simulink model "control"  (R2014b)
settings: Solver=ode45  StartTime=0.0  StopTime=10  RelTol=1e-5  AbsTol=1e-5
values from neighbouring files (symbols this model uses):
  B_eq = 0    [data.m]
  F1 = lqr(A1,B1,Q,R,N)    [data.m]
  F2 = lqr(A2,B2,Q,R,N)    [data.m]
  F3 = lqr(A3,B3,Q,R,N)    [data.m]
  F4 = lqr(A4,B4,Q,R,N)    [data.m]
  F5 = lqr(A5,B5,Q,R,N)    [data.m]
  F6 = lqr(A6,B6,Q,R,N)    [data.m]
  F7 = lqr(A7,B7,Q,R,N)    [data.m]
  F8 = lqr(A8,B8,Q,R,N)    [data.m]
  F9 = lqr(A9,B9,Q,R,N)    [data.m]
  g = 9.81    [data.m]
  initial = pi/2    (= 1.57079632679)    [data.m]
  J_eq = 1.23e-4    (= 0.000123)    [data.m]
  J_p = 1.20e-4    (= 0.00012)    [data.m]
  K_m = K_t    (= 0.028)    [data.m]
  K_t = 0.028    [data.m]
  K_w = 2.3    [data.m]
  l_p = 0.191    [data.m]
  m = 0.027    [data.m]
  r = 0.0826    [data.m]
  R_m = 3.3    [data.m]
libraries: fuzblock x16
settings Model: Creator=Karol  LastModifiedBy=Aramil_2
settings DataIOCC: SignalLoggingSaveFormat=ModelDataLogs
settings OptimizationCC: ExpressionDepthLimit=2147483647
settings DebuggingCC: UnderspecifiedInitializationDetection=Classic  MergeDetectMultiDrivingBlocksExec=none  FcnCallInpInsideContextMsg=UseLocalSettings  StateNameClashWarn=warning
settings GRTTargetCC: CombineOutputUpdateFcns=off  GRTInterface=on

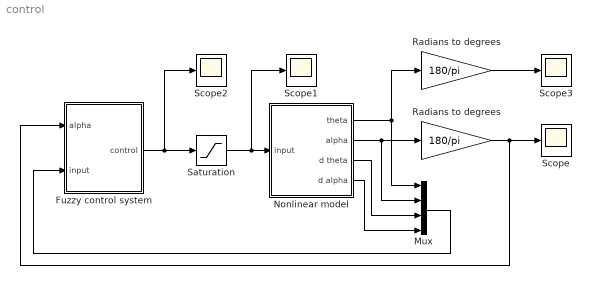
== system control ==
  Fuzzy control system : Subsystem
  Mux : Mux
  "Nonlinear model " : Subsystem
  Radians to degrees : Gain  Gain=180/pi
  "Radians to degrees " : Gain  Gain=180/pi
  Saturation : Saturate  UpperLimit=10  LowerLimit=-10
  Scope{,1..3} (4 alike) : Scope
      Scope settings: YMin=220  YMax=360
      Scope1 settings: TimeRange=20  YMin=0.5375  YMax=0.585
      Scope2 settings: YMin=0.5375  YMax=0.585  SaveName=ScopeData2
      Scope3 settings: TimeRange=5  SaveName=ScopeData3
  wires:
  "Nonlinear model "/2(alpha) -> "Radians to degrees "/1, Mux/2
  "Radians to degrees "/1 -> Scope/1, Fuzzy control system/1(alpha)
  "Nonlinear model "/1(theta) -> Radians to degrees/1, Mux/1
  Mux/1 -> Fuzzy control system/2(input)
  Fuzzy control system/1(control) -> Scope2/1, Saturation/1
  Saturation/1 -> "Nonlinear model "/1(input), Scope1/1
  Radians to degrees/1 -> Scope3/1
  "Nonlinear model "/3(d theta) -> Mux/3
  "Nonlinear model "/4(d alpha) -> Mux/4

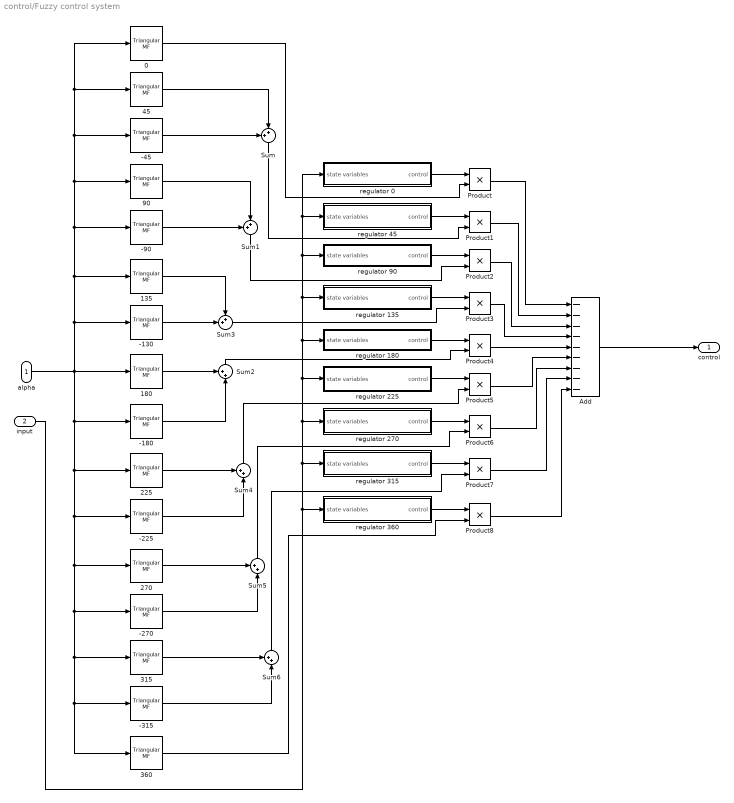
== system control/Fuzzy control system ==
  alpha : Inport
  input : Inport  Port=2
  -130 : fuzblock/Membership  Functions/Triangular MF  a=-180  b=-125  c=-90
  -180 : fuzblock/Membership  Functions/Triangular MF  a=-225  b=-180  c=-130
  -225 : fuzblock/Membership  Functions/Triangular MF  a=-270  b=-225  c=-180
  -270 : fuzblock/Membership  Functions/Triangular MF  a=-315  b=-270  c=-225
  -315 : fuzblock/Membership  Functions/Triangular MF  a=0  b=-315  c=-280
  -45 : fuzblock/Membership  Functions/Triangular MF  a=-90  b=-45  c=0
  -90 : fuzblock/Membership  Functions/Triangular MF  a=-130  b=-90  c=-45
  0 : fuzblock/Membership  Functions/Triangular MF  a=-90  b=0  c=90
  135 : fuzblock/Membership  Functions/Triangular MF  a=90  b=135  c=180
  180 : fuzblock/Membership  Functions/Triangular MF  a=130  b=180  c=225
  225 : fuzblock/Membership  Functions/Triangular MF  a=180  b=225  c=270
  270 : fuzblock/Membership  Functions/Triangular MF  a=225  b=270  c=315
  315 : fuzblock/Membership  Functions/Triangular MF  a=270  b=315  c=360
  360 : fuzblock/Membership  Functions/Triangular MF  a=270  b=360  c=450
  45 : fuzblock/Membership  Functions/Triangular MF  a=0  b=45  c=90
  90 : fuzblock/Membership  Functions/Triangular MF  a=45  b=90  c=130
  Add : Sum  Inputs=---------
  Product{,1..8} (9 alike) : Product  RndMeth=Zero
  Sum{,1..6} (7 alike) : Sum  Inputs=++|
  regulator 0 : Subsystem
  regulator 135 : Subsystem
  regulator 180 : Subsystem
  regulator 225 : Subsystem
  regulator 270 : Subsystem
  regulator 315 : Subsystem
  regulator 360 : Subsystem
  regulator 45 : Subsystem
  regulator 90 : Subsystem
  control : Outport
  wires:
  regulator 0/1(control) -> Product/1
  regulator 45/1(control) -> Product1/1
  regulator 90/1(control) -> Product2/1
  regulator 135/1(control) -> Product3/1
  regulator 180/1(control) -> Product4/1
  regulator 225/1(control) -> Product5/1
  regulator 270/1(control) -> Product6/1
  regulator 315/1(control) -> Product7/1
  regulator 360/1(control) -> Product8/1
  Add/1 -> control/1
  Product/1 -> Add/1
  Product1/1 -> Add/2
  Product2/1 -> Add/3
  Product3/1 -> Add/4
  Product4/1 -> Add/5
  Product5/1 -> Add/6
  Product6/1 -> Add/7
  Product7/1 -> Add/8
  Product8/1 -> Add/9
  0/1 -> Product/2
  Sum/1 -> Product1/2
  Sum1/1 -> Product2/2
  input/1 -> regulator 180/1(state variables), regulator 135/1(state variables), regulator 0/1(state variables), regulator 45/1(state variables), regulator 90/1(state variables), regulator 225/1(state variables), regulator 270/1(state variables), regulator 315/1(state variables), regulator 360/1(state variables)
  45/1 -> Sum/2
  -45/1 -> Sum/1
  90/1 -> Sum1/2
  -90/1 -> Sum1/1
  Sum2/1 -> Product4/2
  Sum3/1 -> Product3/2
  225/1 -> Sum4/1
  -225/1 -> Sum4/2
  315/1 -> Sum6/1
  -315/1 -> Sum6/2
  alpha/1 -> 360/1, -315/1, 315/1, -270/1, 270/1, -225/1, 225/1, -180/1, -90/1, 90/1, 0/1, 45/1, -45/1, 135/1, -130/1, 180/1
  360/1 -> Product8/2
  Sum4/1 -> Product5/2
  Sum5/1 -> Product6/2
  Sum6/1 -> Product7/2
  135/1 -> Sum3/1
  -130/1 -> Sum3/2
  180/1 -> Sum2/1
  -180/1 -> Sum2/2
  270/1 -> Sum5/1
  -270/1 -> Sum5/2

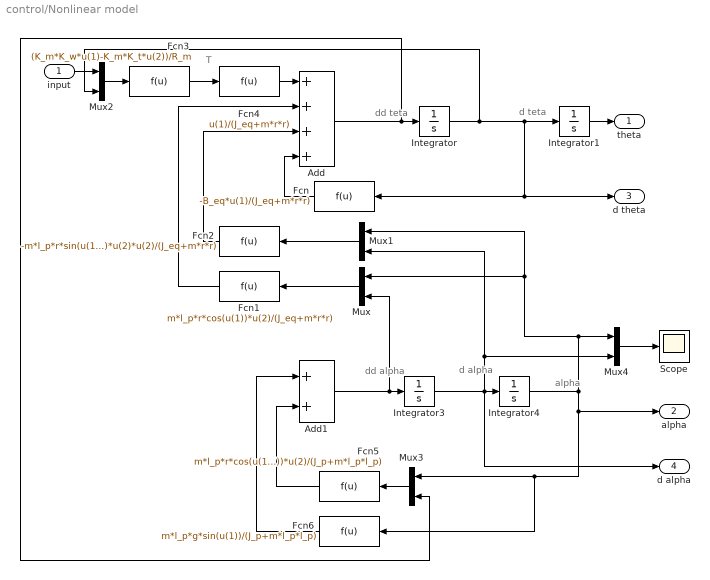
== system control/Nonlinear model  ==
  note: dd teta
  note: d teta
  note: dd alpha
  note: d alpha
  note: alpha
  note: T
  input : Inport
  Add : Sum  Inputs=++++
  Add1 : Sum
  Fcn : Fcn  Expr=-B_eq*u(1)/(J_eq+m*r*r)
  Fcn1 : Fcn  Expr=m*l_p*r*cos(u(1))*u(2)/(J_eq+m*r*r)
  Fcn2 : Fcn  Expr=-m*l_p*r*sin(u(1))*u(2)*u(2)/(J_eq+m*r*r)
  Fcn3 : Fcn  Expr=(K_m*K_w*u(1)-K_m*K_t*u(2))/R_m
  Fcn4 : Fcn  Expr=u(1)/(J_eq+m*r*r)
  Fcn5 : Fcn  Expr=m*l_p*r*cos(u(1))*u(2)/(J_p+m*l_p*l_p)
  Fcn6 : Fcn  Expr=m*l_p*g*sin(u(1))/(J_p+m*l_p*l_p)
  Integrator : Integrator
  Integrator1 : Integrator
  Integrator3 : Integrator
  Integrator4 : Integrator  InitialCondition=initial
  Mux{,1..4} (5 alike) : Mux  Inputs=2
  Scope : Scope
      settings: SaveName=ScopeData7
  theta : Outport
  alpha : Outport  Port=2
  d theta : Outport  Port=3
  d alpha : Outport  Port=4
  wires:
  Add/1 -> Integrator/1, Mux3/2
  Integrator/1 -> Mux2/2, d theta/1, Fcn/1, Integrator1/1
  Add1/1 -> Integrator3/1, Mux/2
  Integrator3/1 -> d alpha/1, Integrator4/1, Mux4/2, Mux1/2
  Integrator4/1 -> Fcn6/1, Mux3/1, alpha/1, Mux/1, Mux1/1, Mux4/1
  Mux/1 -> Fcn1/1
  Mux1/1 -> Fcn2/1
  Mux2/1 -> Fcn3/1
  Fcn3/1 -> Fcn4/1
  Fcn4/1 -> Add/1
  Fcn/1 -> Add/4
  Fcn2/1 -> Add/3
  Fcn1/1 -> Add/2
  Mux3/1 -> Fcn5/1
  Fcn5/1 -> Add1/2
  Fcn6/1 -> Add1/1
  Integrator1/1 -> theta/1
  Mux4/1 -> Scope/1
  input/1 -> Mux2/1

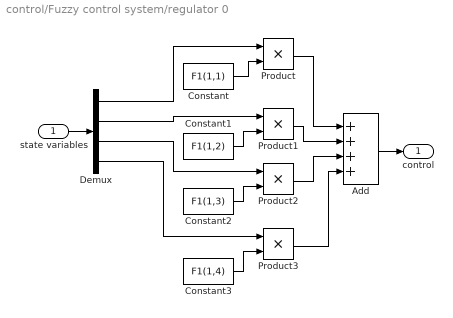
== system control/Fuzzy control system/regulator 0 ==
  state variables : Inport
  Add : Sum  Inputs=++++
  Constant : Constant  Value=F1(1,1)
  Constant1 : Constant  Value=F1(1,2)
  Constant2 : Constant  Value=F1(1,3)
  Constant3 : Constant  Value=F1(1,4)
  Demux : Demux
  Product{,1..3} (4 alike) : Product  RndMeth=Zero
  control : Outport
  wires:
  Demux/1 -> Product/1
  Constant/1 -> Product/2
  Constant1/1 -> Product1/2
  Demux/2 -> Product1/1
  Constant2/1 -> Product2/2
  Demux/3 -> Product2/1
  Constant3/1 -> Product3/2
  Demux/4 -> Product3/1
  Product/1 -> Add/1
  Product1/1 -> Add/2
  Product2/1 -> Add/3
  Product3/1 -> Add/4
  state variables/1 -> Demux/1
  Add/1 -> control/1

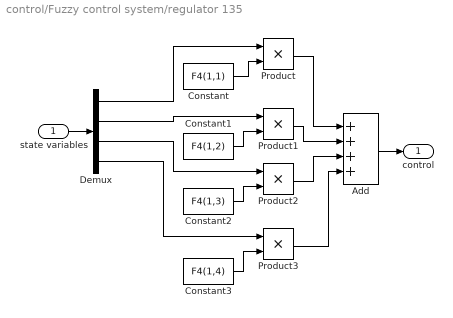
== system control/Fuzzy control system/regulator 135 ==
  state variables : Inport
  Add : Sum  Inputs=++++
  Constant : Constant  Value=F4(1,1)
  Constant1 : Constant  Value=F4(1,2)
  Constant2 : Constant  Value=F4(1,3)
  Constant3 : Constant  Value=F4(1,4)
  Demux : Demux
  Product{,1..3} (4 alike) : Product  RndMeth=Zero
  control : Outport
  wires:
  Add/1 -> control/1
  state variables/1 -> Demux/1
  Product3/1 -> Add/4
  Product2/1 -> Add/3
  Product1/1 -> Add/2
  Product/1 -> Add/1
  Demux/4 -> Product3/1
  Constant3/1 -> Product3/2
  Demux/3 -> Product2/1
  Constant2/1 -> Product2/2
  Demux/2 -> Product1/1
  Constant1/1 -> Product1/2
  Constant/1 -> Product/2
  Demux/1 -> Product/1

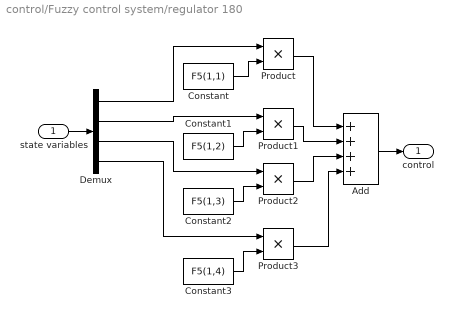
== system control/Fuzzy control system/regulator 180 ==
  state variables : Inport
  Add : Sum  Inputs=++++
  Constant : Constant  Value=F5(1,1)
  Constant1 : Constant  Value=F5(1,2)
  Constant2 : Constant  Value=F5(1,3)
  Constant3 : Constant  Value=F5(1,4)
  Demux : Demux
  Product{,1..3} (4 alike) : Product  RndMeth=Zero
  control : Outport
  wires:
  Demux/1 -> Product/1
  Constant/1 -> Product/2
  Constant1/1 -> Product1/2
  Demux/2 -> Product1/1
  Constant2/1 -> Product2/2
  Demux/3 -> Product2/1
  Constant3/1 -> Product3/2
  Demux/4 -> Product3/1
  Product/1 -> Add/1
  Product1/1 -> Add/2
  Product2/1 -> Add/3
  Product3/1 -> Add/4
  state variables/1 -> Demux/1
  Add/1 -> control/1

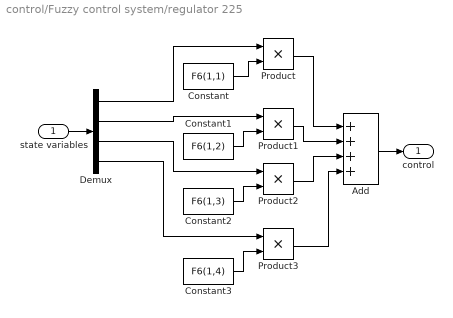
== system control/Fuzzy control system/regulator 225 ==
  state variables : Inport
  Add : Sum  Inputs=++++
  Constant : Constant  Value=F6(1,1)
  Constant1 : Constant  Value=F6(1,2)
  Constant2 : Constant  Value=F6(1,3)
  Constant3 : Constant  Value=F6(1,4)
  Demux : Demux
  Product{,1..3} (4 alike) : Product  RndMeth=Zero
  control : Outport
  wires:
  Add/1 -> control/1
  state variables/1 -> Demux/1
  Product3/1 -> Add/4
  Product2/1 -> Add/3
  Product1/1 -> Add/2
  Product/1 -> Add/1
  Demux/4 -> Product3/1
  Constant3/1 -> Product3/2
  Demux/3 -> Product2/1
  Constant2/1 -> Product2/2
  Demux/2 -> Product1/1
  Constant1/1 -> Product1/2
  Constant/1 -> Product/2
  Demux/1 -> Product/1

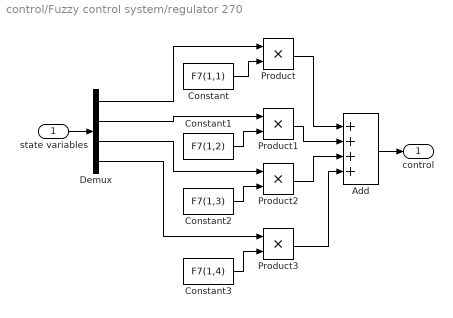
== system control/Fuzzy control system/regulator 270 ==
  state variables : Inport
  Add : Sum  Inputs=++++
  Constant : Constant  Value=F7(1,1)
  Constant1 : Constant  Value=F7(1,2)
  Constant2 : Constant  Value=F7(1,3)
  Constant3 : Constant  Value=F7(1,4)
  Demux : Demux
  Product{,1..3} (4 alike) : Product  RndMeth=Zero
  control : Outport
  wires:
  Demux/1 -> Product/1
  Constant/1 -> Product/2
  Constant1/1 -> Product1/2
  Demux/2 -> Product1/1
  Constant2/1 -> Product2/2
  Demux/3 -> Product2/1
  Constant3/1 -> Product3/2
  Demux/4 -> Product3/1
  Product/1 -> Add/1
  Product1/1 -> Add/2
  Product2/1 -> Add/3
  Product3/1 -> Add/4
  state variables/1 -> Demux/1
  Add/1 -> control/1

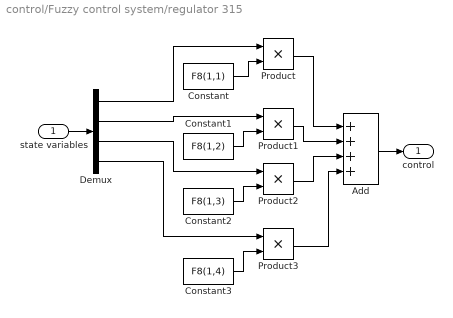
== system control/Fuzzy control system/regulator 315 ==
  state variables : Inport
  Add : Sum  Inputs=++++
  Constant : Constant  Value=F8(1,1)
  Constant1 : Constant  Value=F8(1,2)
  Constant2 : Constant  Value=F8(1,3)
  Constant3 : Constant  Value=F8(1,4)
  Demux : Demux
  Product{,1..3} (4 alike) : Product  RndMeth=Zero
  control : Outport
  wires:
  Add/1 -> control/1
  state variables/1 -> Demux/1
  Product3/1 -> Add/4
  Product2/1 -> Add/3
  Product1/1 -> Add/2
  Product/1 -> Add/1
  Demux/4 -> Product3/1
  Constant3/1 -> Product3/2
  Demux/3 -> Product2/1
  Constant2/1 -> Product2/2
  Demux/2 -> Product1/1
  Constant1/1 -> Product1/2
  Constant/1 -> Product/2
  Demux/1 -> Product/1

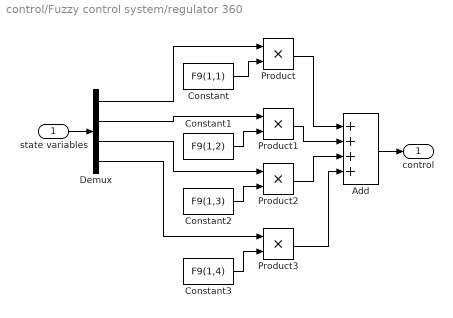
== system control/Fuzzy control system/regulator 360 ==
  state variables : Inport
  Add : Sum  Inputs=++++
  Constant : Constant  Value=F9(1,1)
  Constant1 : Constant  Value=F9(1,2)
  Constant2 : Constant  Value=F9(1,3)
  Constant3 : Constant  Value=F9(1,4)
  Demux : Demux
  Product{,1..3} (4 alike) : Product  RndMeth=Zero
  control : Outport
  wires:
  Demux/1 -> Product/1
  Constant/1 -> Product/2
  Constant1/1 -> Product1/2
  Demux/2 -> Product1/1
  Constant2/1 -> Product2/2
  Demux/3 -> Product2/1
  Constant3/1 -> Product3/2
  Demux/4 -> Product3/1
  Product/1 -> Add/1
  Product1/1 -> Add/2
  Product2/1 -> Add/3
  Product3/1 -> Add/4
  state variables/1 -> Demux/1
  Add/1 -> control/1

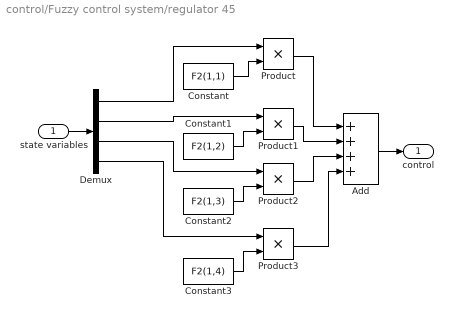
== system control/Fuzzy control system/regulator 45 ==
  state variables : Inport
  Add : Sum  Inputs=++++
  Constant : Constant  Value=F2(1,1)
  Constant1 : Constant  Value=F2(1,2)
  Constant2 : Constant  Value=F2(1,3)
  Constant3 : Constant  Value=F2(1,4)
  Demux : Demux
  Product{,1..3} (4 alike) : Product  RndMeth=Zero
  control : Outport
  wires:
  Add/1 -> control/1
  state variables/1 -> Demux/1
  Product3/1 -> Add/4
  Product2/1 -> Add/3
  Product1/1 -> Add/2
  Product/1 -> Add/1
  Demux/4 -> Product3/1
  Constant3/1 -> Product3/2
  Demux/3 -> Product2/1
  Constant2/1 -> Product2/2
  Demux/2 -> Product1/1
  Constant1/1 -> Product1/2
  Constant/1 -> Product/2
  Demux/1 -> Product/1

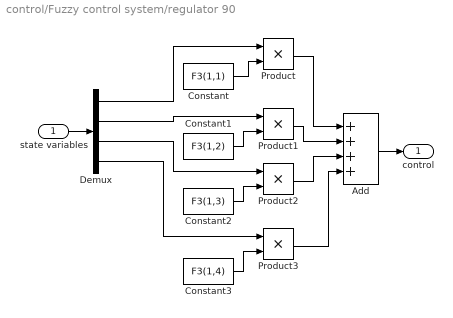
== system control/Fuzzy control system/regulator 90 ==
  state variables : Inport
  Add : Sum  Inputs=++++
  Constant : Constant  Value=F3(1,1)
  Constant1 : Constant  Value=F3(1,2)
  Constant2 : Constant  Value=F3(1,3)
  Constant3 : Constant  Value=F3(1,4)
  Demux : Demux
  Product{,1..3} (4 alike) : Product  RndMeth=Zero
  control : Outport
  wires:
  Demux/1 -> Product/1
  Constant/1 -> Product/2
  Constant1/1 -> Product1/2
  Demux/2 -> Product1/1
  Constant2/1 -> Product2/2
  Demux/3 -> Product2/1
  Constant3/1 -> Product3/2
  Demux/4 -> Product3/1
  Product/1 -> Add/1
  Product1/1 -> Add/2
  Product2/1 -> Add/3
  Product3/1 -> Add/4
  state variables/1 -> Demux/1
  Add/1 -> control/1
